simulink model "Im_shema2"  (Simulink 5.0)
settings: Solver=ode45  StartTime=0.0  StopTime=17.0  RelTol=1e-3
libraries: dspsigops x4
settings Model: LastModifiedBy=Agressor

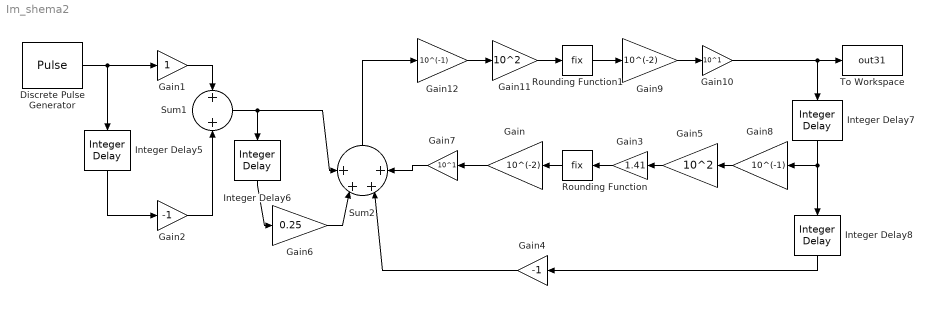
== system Im_shema2 ==
  Discrete Pulse Generator : DiscretePulseGenerator  Period=10000
  Gain : Gain  Orientation=left  Gain=10^(-2)  SaturateOnIntegerOverflow=on
  Gain1 : Gain  SaturateOnIntegerOverflow=on
  Gain10 : Gain  Gain=10^1  SaturateOnIntegerOverflow=on
  Gain11 : Gain  Gain=10^2  SaturateOnIntegerOverflow=on
  Gain12 : Gain  Gain=10^(-1)  SaturateOnIntegerOverflow=on
  Gain2 : Gain  Gain=-1  SaturateOnIntegerOverflow=on
  Gain3 : Gain  Orientation=left  Gain=1.41  SaturateOnIntegerOverflow=on
  Gain4 : Gain  Orientation=left  Gain=-1  SaturateOnIntegerOverflow=on
  Gain5 : Gain  Orientation=left  Gain=10^2  SaturateOnIntegerOverflow=on
  Gain6 : Gain  Gain=0.25  SaturateOnIntegerOverflow=on
  Gain7 : Gain  Orientation=left  Gain=10^1  SaturateOnIntegerOverflow=on
  Gain8 : Gain  Orientation=left  Gain=10^(-1)  SaturateOnIntegerOverflow=on
  Gain9 : Gain  Gain=10^(-2)  SaturateOnIntegerOverflow=on
  Integer Delay5 : dspsigops/Integer Delay  Orientation=down  delay=8  ic=0  reset_popup=None
  Integer Delay6 : dspsigops/Integer Delay  Orientation=down  delay=1  ic=0  reset_popup=None
  Integer Delay7 : dspsigops/Integer Delay  Orientation=down  delay=1  ic=0  reset_popup=None
  Integer Delay8 : dspsigops/Integer Delay  Orientation=down  delay=1  ic=0  reset_popup=None
  Rounding Function : Rounding  Orientation=left  Operator=fix
  Rounding Function1 : Rounding  Operator=fix
  Sum1 : Sum  Inputs=2  SaturateOnIntegerOverflow=on  InputSameDT=on
  Sum2 : Sum  Orientation=up  Inputs=4  SaturateOnIntegerOverflow=on  InputSameDT=on
  To Workspace : ToWorkspace  VariableName=out31  SampleTime=-1  SaveFormat=Array
  wires:
  Gain1/1 -> Sum1/1
  Integer Delay5/1 -> Gain2/1
  Gain2/1 -> Sum1/2
  Integer Delay6/1 -> Gain6/1
  Integer Delay8/1 -> Gain4/1
  Discrete Pulse Generator/1 -> Gain1/1, Integer Delay5/1
  Gain/1 -> Gain7/1
  Gain8/1 -> Gain5/1
  Integer Delay7/1 -> Integer Delay8/1, Gain8/1
  Sum2/1 -> Gain12/1
  Gain12/1 -> Gain11/1
  Gain11/1 -> Rounding Function1/1
  Rounding Function1/1 -> Gain9/1
  Gain9/1 -> Gain10/1
  Gain10/1 -> To Workspace/1, Integer Delay7/1
  Gain5/1 -> Gain3/1
  Gain3/1 -> Rounding Function/1
  Rounding Function/1 -> Gain/1
  Sum1/1 -> Sum2/1, Integer Delay6/1
  Gain7/1 -> Sum2/4
  Gain6/1 -> Sum2/2
  Gain4/1 -> Sum2/3
